simulink model "solar_PV"  (R2023b)
settings: Solver=VariableStepAuto  StartTime=0.0  StopTime=10  RelTol=1e-3
libraries: ee_lib x48, nesl_utility x28, fl_lib x4, simulink x1
settings Model: Creator=Akhil Reddy  LastModifiedBy=Akhil Reddy

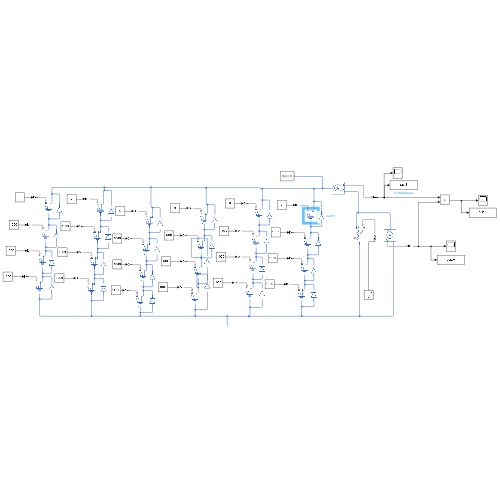
[thumbnail: Simulink's stored preview of the top-level diagram]
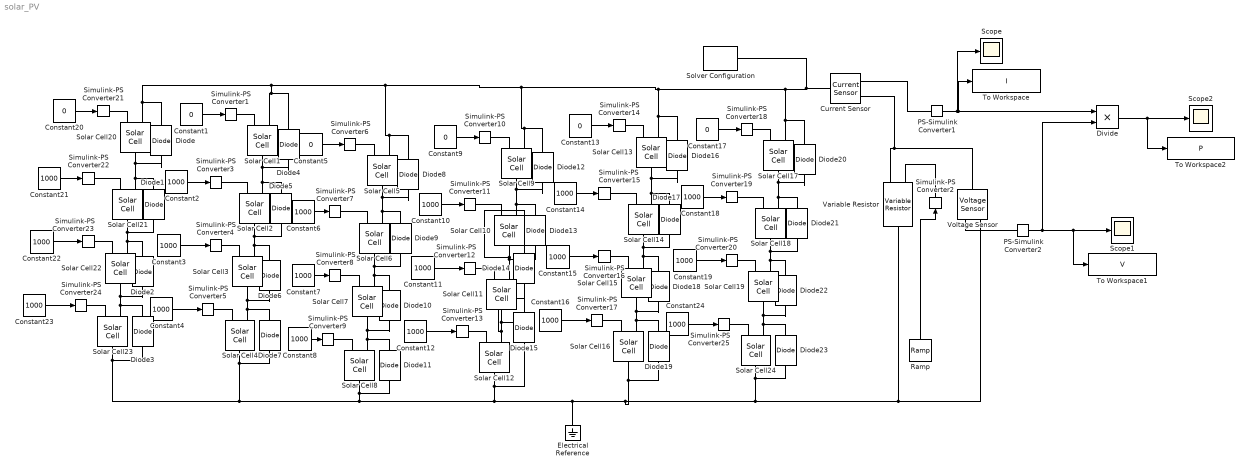
== system solar_PV ==
  Constant{1,5,9,13,17,20} (6 alike) : Constant  Value=0
  Constant{2..4,6..8,10..12,14..16,18..19,21..24} (18 alike) : Constant  Value=1000
  Current Sensor : fl_lib/Electrical/Electrical Sensors/Current Sensor
  Diode{,1..23} (24 alike) : ee_lib/Semiconductors & Converters/Diode  ModelType=ee.enum.diode.modelType.pwl  TableType=ee.enum.diode.tableType.IfMat  IfMat=[.07, .12, .19, 1.75, 4.24, 7.32, 11.2; .16, .3, .72, 2.14, 5.02, 8.35, 13.12] A  VfMat=[.9, 1.15, 1.25, 1.5, 1.75, 2.17, 2.6, 2.85; .58, .68, .75, 1.1, 1.38, 1.77, 2.27, 2.7] V  TjVec=[25, 125] degC  VfVec=[.5, .7, .9, 1.3, 1.7, 2.1, 2.5] V  IfVec=[.1, .2, .5, 1, 2, 4, 7, 10] A  Vf=0.6 V  Ron=0.3 Ohm  Goff=1e-8 S  prmExp=ee.enum.diode.expParam.useTwo  I12=[.0137, .545] A  V12=[.6, .7] V  RS=0 Ohm  Tmeas=25 degC  IS=1e-12 A  ec=1  I1=0.0137 A  V1=0.6 V  N_series=1  N_parallel=1  ZenerEnable=false  Rz=0.3 Ohm  BV=inf V  C_param=ee.enum.diode.capParam.fixed  CJ=0 pF  CJ0=5 pF  Vvec=[.1, 10, 100] V  Cvec=[3.5, 1, .4] pF  VJ=1 V  Mgrad=0.5  FC=0.5  Q_param=ee.enum.diode.recoveryParam.off  iRM=-7.15 A  iF=4 A  didt=-750 A/us  trr_factor=3  trr=115 ns  Qrr=150 nA*s  Vr=-600 V  Ls=150 nH  Erec=0.03 J  TT=50 ns  tau=100 ns  T_param=ee.enum.diode.temperatureParam.off  Tdevice=25 degC  I1_T2=0.245 A  V1_T2=0.5 V  IS_T2=1.25e-7 A  Tmeas2=125 degC  XTI_param=ee.enum.diode.xtiParam.pn  XTI=3  EG_param=ee.enum.diode.egapParam.material_si  EG=1.11 eV  dBVdT=0 V/K  enable_faults=simscape.enum.onoff.off  fault_action=simscape.enum.assert.action.none  fault_types=ee.enum.diode.faults.open  tau_fault=1e-3 s  IfMat_faulted=[.07, .12, .19, 1.75, 4.24, 7.32, 11.2; .16, .3, .72, 2.14, 4.02, 6.35, 9.12] A  VfMat_faulted=[.9, 1.15, 1.25, 1.5, 1.75, 2.17, 2.6, 2.85; .58, .68, .75, 1.1, 1.38, 1.77, 2.27, 2.7] V  VfVec_faulted=[.5, .7, .9, 1.3, 1.7, 2.1, 2.5] V  IfVec_faulted=[.1, .2, .5, 1, 2, 4, 7, 10] A  Ropen_faulted=1000 Ohm  Gshort_faulted=1000 1/Ohm  Vf_faulted=0.6 V  Ron_faulted=0.3 Ohm  Goff_faulted=1e-8 S  I12_faulted=[.0137, .545] A  V12_faulted=[.6, .7] V  IS_faulted=1e-12 A  ec_faulted=1  I1_faulted=0.0137 A  V1_faulted=0.6 V  RS_faulted=0 Ohm  Rz_faulted=0.3 Ohm  BV_faulted=inf V  Cscale_faulted=100  fault_trigger=ee.enum.faults.faultTrigger.temporal  t_fault=inf s  max_permissible_voltage=inf V  n_fail_on_voltage=1  max_permissible_current=inf A  t_fail_on_current=1 s  max_permissible_dVdt=inf V/s  enable_fault_input=simscape.enum.onoff.off  i_specify=off  i_priority=None  i=0 A  i_nominal_specify=off  i_nominal_unit=A  i_nominal_value=1  v_specify=off  v_priority=None  v=0 V  v_nominal_specify=off  v_nominal_unit=V  v_nominal_value=1  v_capacitor_specify=off  v_capacitor_priority=None  v_capacitor=0 V  v_capacitor_nominal_specify=off  v_capacitor_nominal_unit=V  v_capacitor_nominal_value=1  faulted_specify=off  faulted_priority=None  faulted=0  faulted_nominal_specify=off  faulted_nominal_unit=1  faulted_nominal_value=1  i_diode_specify=off  i_diode_priority=None  i_diode=0 A  i_diode_nominal_specify=off  i_diode_nominal_unit=A  i_diode_nominal_value=1  v_diode_specify=off  v_diode_priority=None  v_diode=0 V  v_diode_nominal_specify=off  v_diode_nominal_unit=V  v_diode_nominal_value=1  i_capacitor_specify=off  i_capacitor_priority=None  i_capacitor=0 A  i_capacitor_nominal_specify=off  i_capacitor_nominal_unit=A  i_capacitor_nominal_value=1  power_dissipated_specify=off  power_dissipated_priority=None  power_dissipated=0 W  power_dissipated_nominal_specify=off  power_dissipated_nominal_unit=W  power_dissipated_nominal_value=1  fidelity_level=ee.enum.diode.fidelity.includeChargeDyn  rec_loss_model=ee.enum.diode.reverseRecoveryModel.fixed  ErecVal=0 J  scaleWithIandV=true  ErecMat=zeros(2, 3) J  TjrecVec=[298.15, 398.15] K  IfrecVec=[.1, 1, 10] A  IrecVal=10 A  VrecVal=10 V  tFilter=1 / 1000 / 100 s  max_permissible_temperature=inf K  t_fail_on_temperature=1 s  thermal_network_parameterization=ee.enum.thermalNetworkTopology.junctionCase  Rth=[0, 10] K/W  Rth_Cauer=[1, 3, 10] K/W  Rth_Foster=[4, 6] K/W  thermal_mass_parameterization=ee.enum.thermalNetwork.timeconstant  thermal_mass=[0, 1] J/K  thermal_mass_Cauer=[.1, .3, 1] J/K  thermal_mass_Foster=[1.5, 3] J/K  thermal_time_constant=[0, 10] s  thermal_time_constant_Cauer=[1, 3, 10] s  thermal_time_constant_Foster=[6, 18] s  thermal_mass_initial_temperatures=[25, 25] degC  thermal_mass_initial_temperatures_Cauer=[25, 25, 25] degC  junction_thermal_mass=0.01 J/K  Tvec_initial_Foster=[25, 25, 25, 25] degC  no_thermal_network=0  junction_temperature_specify=off  junction_temperature_priority=None  junction_temperature=25 degC  junction_temperature_nominal_specify=off  junction_temperature_nominal_unit=degC  junction_temperature_nominal_value=1
  Divide : Product
  Electrical Reference : fl_lib/Electrical/Electrical Elements/Electrical Reference
  PS-Simulink Converter1 : nesl_utility/PS-Simulink Converter  PhysicalDomain=network_engine_domain  SubClassName=ps_output  LeftPortType=input  RightPortType=output  PseudoPeriodic=off  Frequencies=[]  VectorFormat=inherit  Unit=inherit  AffineConversion=off
  PS-Simulink Converter2 : nesl_utility/PS-Simulink Converter  PhysicalDomain=network_engine_domain  SubClassName=ps_output  LeftPortType=input  RightPortType=output  PseudoPeriodic=off  Frequencies=[]  VectorFormat=inherit  Unit=inherit  AffineConversion=off
  Ramp : simulink/Sources/Ramp  slope=4 * 53.77 * 6  start=0  InitialOutput=0
  Scope : Scope
  Scope1 : Scope
  Scope2 : Scope
  Simulink-PS Converter{1..25} (25 alike) : nesl_utility/Simulink-PS Converter  PhysicalDomain=network_engine_domain  SubClassName=ps_input  LeftPortType=input  RightPortType=output  PseudoPeriodic=off  Frequencies=[]  NoiseDistribution=none  NoiseParameters=[]  Unit=1  AffineConversion=off  FilteringAndDerivatives=provide  SimscapeFilterOrder=1  InputFilterTimeConstant=0.001  UdotUserProvided=0
  Solar Cell{1..24} (24 alike) : ee_lib/Sources/Solar Cell  prm=1  Isc=2.28 A  Voc=2.242 V  Is=1e-6 A  Is2=0 A  Iph=7.34 A  Ir0=1000 W/m^2  ec=1.5  N2=2  Rs=0.001 Ohm  Rp=inf Ohm  N_series=160  N_parallel=6  TIPH1=0.045 1/K  EG=1.11 eV  TXIS1=3  TXIS2=3  TRS1=0  TRP1=0  Tmeas=25 degC  TFIXED=25 degC  thermal_mass=100 J/K  initial_temperature=25 degC
  Solver Configuration : nesl_utility/Solver Configuration  PhysicalDomain=network_engine_domain  SubClassName=solver  LeftPortType=input  RightPortType=generic  Tones=[]  Harmonics=[]  SimulateNoise=off  Profile=off  UseLocalSampling=off  EnableSwitchedLinearOptims=on  FrequencyDomain=off  UseCCode=off  RelTol=0.001  AbsTol=0.001  MinStep=1e-09  ToWorkspace=off  RevertToSquareIcSolve=off  NumHomotopyIterations=100  PhasorMode=off  PhasorModeNumHarmonics=1  ConsistencySolver=NEWTON_XTOL_AFTER_FTOL  IndexReductionMethod=DerivativeReplacement  DoDC=off  ResidualTolerance=1e-09  ConsistencyTolSource=GLOBAL  ConsistencyAbsTol=0.001  ConsistencyRelTol=0.001  ConsistencyTolFactor=0.001  UseLocalSolver=off  LocalSolverChoice=NE_BACKWARD_EULER_ADVANCER  ResolveIndetEquations=on  FunctionEvalNumThread=1  LocalSolverSampleTime=0.001  DoFixedCost=off  MaxNonlinIter=3  MaxModeIter=2  ComputeImpulses=off  ImpulseIterations=2  LinearAlgebra=auto  LinearAlgebraNumThread=0  EquationFormulation=NE_TIME_EF  DelaysMemoryBudget=1024  AutomaticFiltering=on  FilteringTimeConstant=0.001  PartitionStorageMethod=AS_NEEDED  PartitionMemoryBudget=1024  PartitionMethod=ROBUST  MultibodyUseLocalSolver=off  MultibodyLocalSolverChoice=ODE1  MultibodyLocalSolverSampleTime=0.001
  To Workspace : ToWorkspace  VariableName=I  SaveFormat=Structure With Time  SampleTime=-1
  To Workspace1 : ToWorkspace  VariableName=V  SaveFormat=Structure With Time  SampleTime=-1
  To Workspace2 : ToWorkspace  VariableName=P  SaveFormat=Structure With Time  SampleTime=-1
  Variable Resistor : fl_lib/Electrical/Electrical Elements/Variable Resistor  Rmin=0 Ohm  thermalEnable=false  thermal_mass=1 J/K  i_specify=off  i_priority=None  i=0 A  i_nominal_specify=off  i_nominal_unit=A  i_nominal_value=1  v_specify=off  v_priority=None  v=0 V  v_nominal_specify=off  v_nominal_unit=V  v_nominal_value=1  T_specify=off  T_priority=None  T=300 K  T_nominal_specify=off  T_nominal_unit=K  T_nominal_value=1
  Voltage Sensor : fl_lib/Electrical/Electrical Sensors/Voltage Sensor
  wires:
  PS-Simulink Converter1/1 -> Divide/1, To Workspace/1, Scope/1
  Ramp/1 -> Simulink-PS Converter2/1
  PS-Simulink Converter2/1 -> Divide/2, To Workspace1/1, Scope1/1
  Divide/1 -> Scope2/1, To Workspace2/1
  Constant23/1 -> Simulink-PS Converter24/1
  Constant20/1 -> Simulink-PS Converter21/1
  Constant21/1 -> Simulink-PS Converter22/1
  Constant22/1 -> Simulink-PS Converter23/1
  Constant1/1 -> Simulink-PS Converter1/1
  Constant3/1 -> Simulink-PS Converter4/1
  Constant2/1 -> Simulink-PS Converter3/1
  Constant4/1 -> Simulink-PS Converter5/1
  Constant5/1 -> Simulink-PS Converter6/1
  Constant7/1 -> Simulink-PS Converter8/1
  Constant6/1 -> Simulink-PS Converter7/1
  Constant8/1 -> Simulink-PS Converter9/1
  Constant9/1 -> Simulink-PS Converter10/1
  Constant11/1 -> Simulink-PS Converter12/1
  Constant10/1 -> Simulink-PS Converter11/1
  Constant12/1 -> Simulink-PS Converter13/1
  Constant13/1 -> Simulink-PS Converter14/1
  Constant15/1 -> Simulink-PS Converter16/1
  Constant14/1 -> Simulink-PS Converter15/1
  Constant16/1 -> Simulink-PS Converter17/1
  Constant17/1 -> Simulink-PS Converter18/1
  Constant19/1 -> Simulink-PS Converter20/1
  Constant18/1 -> Simulink-PS Converter19/1
  Constant24/1 -> Simulink-PS Converter25/1
  connections:
  Variable Resistor/LConn2 -- Voltage Sensor/LConn1 -- Current Sensor/RConn2
  PS-Simulink Converter1/LConn1 -- Current Sensor/RConn1
  Simulink-PS Converter2/RConn1 -- Variable Resistor/LConn1
  Voltage Sensor/RConn1 -- PS-Simulink Converter2/LConn1
  Solar Cell23/LConn1 -- Simulink-PS Converter24/RConn1
  Solar Cell22/LConn1 -- Simulink-PS Converter23/RConn1
  Solar Cell21/LConn1 -- Simulink-PS Converter22/RConn1
  Solar Cell21/LConn2 -- Diode1/RConn1 -- Diode/LConn1 -- Solar Cell20/RConn1
  Solar Cell22/RConn1 -- Diode2/LConn1 -- Diode3/RConn1 -- Solar Cell23/LConn2
  Solar Cell21/RConn1 -- Diode1/LConn1 -- Diode2/RConn1 -- Solar Cell22/LConn2
  Solar Cell20/LConn1 -- Simulink-PS Converter21/RConn1
  Solar Cell17/LConn2 -- Current Sensor/LConn1 -- Solver Configuration/RConn1 -- Diode16/RConn1 -- Solar Cell13/LConn2 -- Diode12/RConn1 -- Solar Cell9/LConn2 -- Diode8/RConn1 -- Solar Cell5/LConn2 -- Solar Cell1/LConn2 -- Diode4/RConn1 -- Diode/RConn1 -- Solar Cell20/LConn2 -- Diode20/RConn1
  Solar Cell24/RConn1 -- Electrical Reference/LConn1 -- Diode15/LConn1 -- Solar Cell12/RConn1 -- Diode11/LConn1 -- Solar Cell8/RConn1 -- Diode7/LConn1 -- Solar Cell4/RConn1 -- Diode3/LConn1 -- Solar Cell23/RConn1 -- Diode19/LConn1 -- Solar Cell16/RConn1 -- Voltage Sensor/RConn2 -- Variable Resistor/RConn1 -- Diode23/LConn1
  Solar Cell3/LConn2 -- Diode6/RConn1 -- Diode5/LConn1 -- Solar Cell2/RConn1
  Solar Cell4/LConn2 -- Diode7/RConn1 -- Diode6/LConn1 -- Solar Cell3/RConn1
  Solar Cell1/RConn1 -- Diode4/LConn1 -- Diode5/RConn1 -- Solar Cell2/LConn2
  Solar Cell2/LConn1 -- Simulink-PS Converter3/RConn1
  Solar Cell3/LConn1 -- Simulink-PS Converter4/RConn1
  Solar Cell4/LConn1 -- Simulink-PS Converter5/RConn1
  Solar Cell1/LConn1 -- Simulink-PS Converter1/RConn1
  Solar Cell7/LConn2 -- Diode10/RConn1 -- Diode9/LConn1 -- Solar Cell6/RConn1
  Solar Cell8/LConn2 -- Diode11/RConn1 -- Diode10/LConn1 -- Solar Cell7/RConn1
  Solar Cell5/RConn1 -- Diode8/LConn1 -- Diode9/RConn1 -- Solar Cell6/LConn2
  Solar Cell6/LConn1 -- Simulink-PS Converter7/RConn1
  Solar Cell7/LConn1 -- Simulink-PS Converter8/RConn1
  Solar Cell8/LConn1 -- Simulink-PS Converter9/RConn1
  Solar Cell5/LConn1 -- Simulink-PS Converter6/RConn1
  Diode14/RConn1 -- Solar Cell11/LConn2 -- Diode13/LConn1 -- Solar Cell10/RConn1
  Solar Cell12/LConn2 -- Diode15/RConn1 -- Diode14/LConn1 -- Solar Cell11/RConn1
  Solar Cell9/RConn1 -- Diode12/LConn1 -- Diode13/RConn1 -- Solar Cell10/LConn2
  Solar Cell10/LConn1 -- Simulink-PS Converter11/RConn1
  Solar Cell11/LConn1 -- Simulink-PS Converter12/RConn1
  Solar Cell12/LConn1 -- Simulink-PS Converter13/RConn1
  Solar Cell9/LConn1 -- Simulink-PS Converter10/RConn1
  Solar Cell15/LConn2 -- Diode18/RConn1 -- Diode17/LConn1 -- Solar Cell14/RConn1
  Solar Cell16/LConn2 -- Diode19/RConn1 -- Diode18/LConn1 -- Solar Cell15/RConn1
  Solar Cell13/RConn1 -- Diode16/LConn1 -- Diode17/RConn1 -- Solar Cell14/LConn2
  Solar Cell14/LConn1 -- Simulink-PS Converter15/RConn1
  Solar Cell15/LConn1 -- Simulink-PS Converter16/RConn1
  Solar Cell16/LConn1 -- Simulink-PS Converter17/RConn1
  Solar Cell13/LConn1 -- Simulink-PS Converter14/RConn1
  Solar Cell19/LConn2 -- Diode22/RConn1 -- Diode21/LConn1 -- Solar Cell18/RConn1
  Solar Cell24/LConn2 -- Diode23/RConn1 -- Diode22/LConn1 -- Solar Cell19/RConn1
  Solar Cell17/RConn1 -- Diode20/LConn1 -- Diode21/RConn1 -- Solar Cell18/LConn2
  Solar Cell18/LConn1 -- Simulink-PS Converter19/RConn1
  Solar Cell19/LConn1 -- Simulink-PS Converter20/RConn1
  Solar Cell24/LConn1 -- Simulink-PS Converter25/RConn1
  Solar Cell17/LConn1 -- Simulink-PS Converter18/RConn1
